simulink model "activationFunction"  (R2018a)
settings: Solver=FixedStepAuto  StartTime=0.0  StopTime=50  FixedStep=1/1000  RelTol=1e-3
undefined symbols (not defined in the file): DiscIntNeverNeededParam
settings Model: Creator=wout7  LastModifiedBy=wout7

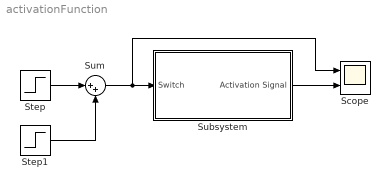
== system activationFunction ==
  Scope : Scope  NumInputPorts=2
  Step : Step  Time=5  SampleTime=0
  Step1 : Step  Time=30  After=-1  SampleTime=0
  Subsystem : Subsystem
  Sum : Sum  Inputs=|++
  wires:
  Subsystem/1(Activation Signal) -> Scope/2
  Step/1 -> Sum/1
  Step1/1 -> Sum/2
  Sum/1 -> Scope/1, Subsystem/1(Switch)

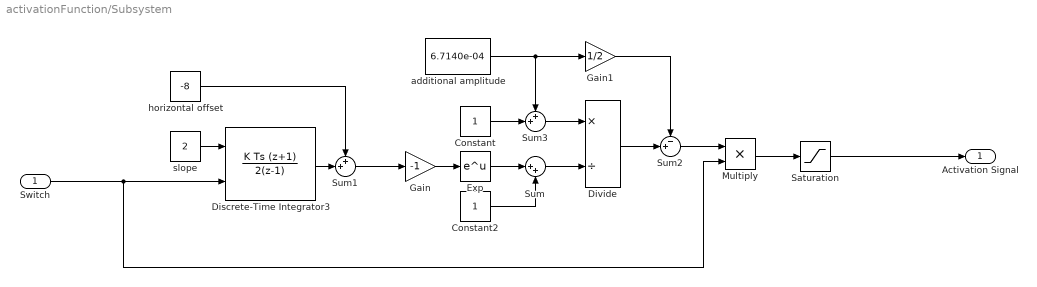
== system activationFunction/Subsystem ==
  Switch : Inport
  Constant : Constant
  Constant2 : Constant
  Discrete-Time Integrator3 : DiscreteIntegrator  IntegratorMethod=Integration: Trapezoidal  ExternalReset=rising  SampleTime=-1  UpperSaturationLimit=1  LowerSaturationLimit=0  ICPrevOutput=DiscIntNeverNeededParam  ICPrevScaledInput=DiscIntNeverNeededParam
  Divide : Product  Inputs=*/
  Exp : Math  SaturateOnIntegerOverflow=on
  Gain : Gain  Gain=-1
  Gain1 : Gain  Gain=1/2
  Multiply : Product
  Saturation : Saturate  UpperLimit=1  LowerLimit=0
  Sum : Sum  Inputs=|++
  Sum1 : Sum  Inputs=++|
  Sum2 : Sum  Inputs=-+|
  Sum3 : Sum  Inputs=++|
  additional amplitude : Constant  Value=6.7140e-04
  horizontal offset : Constant  Value=-8
  slope : Constant  Value=2
  Activation Signal : Outport
  wires:
  Constant/1 -> Sum3/2
  Exp/1 -> Sum/1
  additional amplitude/1 -> Sum3/1, Gain1/1
  Sum1/1 -> Gain/1
  Gain1/1 -> Sum2/1
  Divide/1 -> Sum2/2
  Sum/1 -> Divide/2
  Gain/1 -> Exp/1
  slope/1 -> Discrete-Time Integrator3/1
  Discrete-Time Integrator3/1 -> Sum1/2
  Constant2/1 -> Sum/2
  Sum2/1 -> Multiply/1
  Sum3/1 -> Divide/1
  horizontal offset/1 -> Sum1/1
  Saturation/1 -> Activation Signal/1
  Multiply/1 -> Saturation/1
  Switch/1 -> Multiply/2, Discrete-Time Integrator3/2
